simulink model "Clab2_EyeMovement"  (R2019a)
settings: Solver=VariableStepAuto  StartTime=0.0  StopTime=3  RelTol=1e-10
values from neighbouring files (symbols this model uses):
  k = [3,5,7]    [Clab2.m]
  Wn = [100]    [Clab2.m]
  Z = [.70]    [Clab2.m]
settings Model: Creator=Pranav Maddula  LastModifiedBy=Pranav Maddula

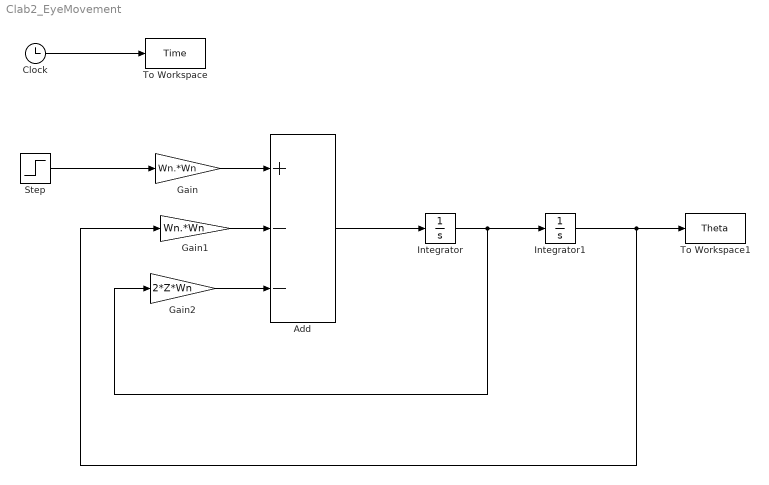
== system Clab2_EyeMovement ==
  Add : Sum  Inputs=+--
  Clock : Clock
  Gain : Gain  Gain=Wn.*Wn
  Gain1 : Gain  Gain=Wn.*Wn
  Gain2 : Gain  Gain=2*Z*Wn
  Integrator : Integrator
  Integrator1 : Integrator
  Step : Step  After=k  SampleTime=0
  To Workspace : ToWorkspace  VariableName=Time  SampleTime=-1
  To Workspace1 : ToWorkspace  VariableName=Theta  SampleTime=-1
  wires:
  Clock/1 -> To Workspace/1
  Step/1 -> Gain/1
  Gain/1 -> Add/1
  Gain2/1 -> Add/3
  Gain1/1 -> Add/2
  Add/1 -> Integrator/1
  Integrator/1 -> Integrator1/1, Gain2/1
  Integrator1/1 -> To Workspace1/1, Gain1/1
